simulink model "main"  (R2016b)
settings: Solver=FixedStepAuto  StartTime=0.0  StopTime=inf  FixedStep=Ts  MaxStep=0.2  RelTol=1e-2
undefined symbols (not defined in the file): checks, datetime, decyear, delta_e, deltae_degrees, deltafl_degrees, deltafr_degrees, deltar_degrees, deltat_1, deltat_2, deltat_3, deltat_4, deltat_5, Earth, F, ft, groundReaction, initialValues, juliandate, LD, leapyear, Light, m, MIL, Newton, Raphson, s, sigbuilder_block, Ts, WGS84
libraries: simulink x68, aerolibutil x17, aerolibtransform2 x15, simulink_extras x13, aerolibasang x5, aerolib6dofsys x5, aerolib6dof2 x4, aerolibwind2 x3, aerolibbdyn x3, vrlib x3, aerolibconvert2 x3, aerolibactuator x2
(part 1 of 10)
settings Model: Creator=Uxío  LastModifiedBy=sork9
settings DataIOCC: ReturnWorkspaceOutputs=on  ReturnWorkspaceOutputsName=spidata
settings OptimizationCC: EfficientMapNaN2IntZero=off  SimCompilerOptimization=on
settings DebuggingCC: ReadBeforeWriteMsg=DisableAll  WriteAfterWriteMsg=DisableAll  WriteAfterReadMsg=DisableAll  MultiTaskDSMMsg=none
settings HardwareCC: TargetBitPerPointer=64  TargetBitPerSizeT=64  TargetBitPerPtrDiffT=64  TargetLongLongMode=on  TargetIntDivRoundTo=Zero  TargetEndianess=LittleEndian  TargetWordSize=64  TargetHWDeviceType=MATLAB Host  ProdEqTarget=off
settings ModelReferenceCC: UpdateModelReferenceTargets=IfOutOfDate
settings SFSimCC: SFSimEcho=off
settings CodeAppCC: MaxIdLength=128
settings GRTTargetCC: TargetLangStandard=C89/C90 (ANSI)  CombineOutputUpdateFcns=off  GRTInterface=on
settings ConfigComp: PSAutoStubLUT=on

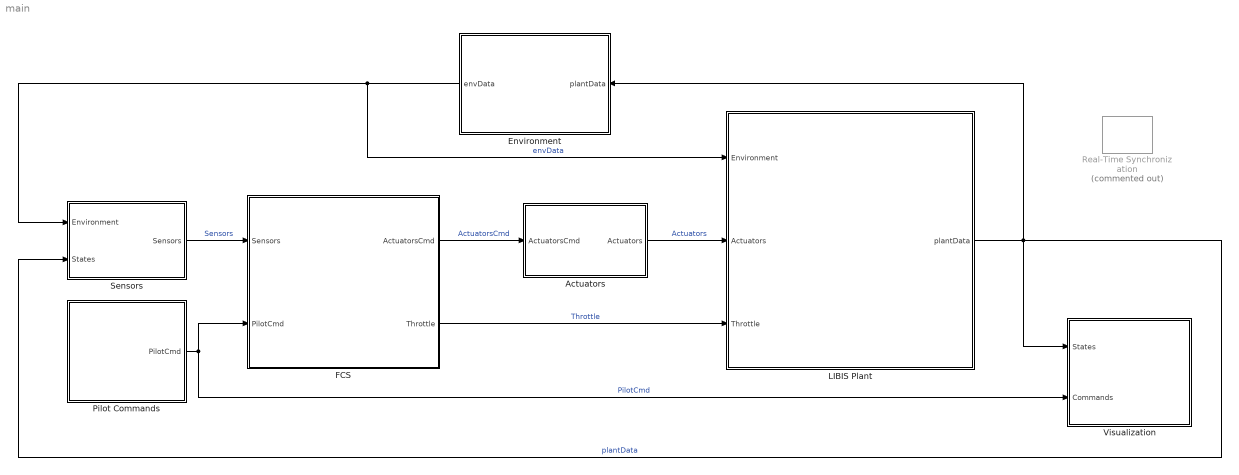
== system main ==
  Actuators : Subsystem  Variant=on
  Environment : Subsystem
      mask Display:
      | imageName='Wind.png';
      | currentPath=get_param(bdroot, 'FileName');
      | positions=strfind(currentPath,'\');
      | imagePath=strcat(currentPath(1:positions(end-1)),'graphics\',imageName);
      | image(imagePath);
  FCS : Subsystem
      mask Display:
      | imageName='FCS.png';
      | currentPath=get_param(bdroot, 'FileName');
      | positions=strfind(currentPath,'\');
      | imagePath=strcat(currentPath(1:positions(end-1)),'graphics\',imageName);
      | image(imagePath);
  LIBIS Plant : Subsystem
      mask Display:
      | imageName='LIBIS_Plant.jpg';
      | currentPath=get_param(bdroot, 'FileName');
      | positions=strfind(currentPath,'\');
      | imagePath=strcat(currentPath(1:positions(end-1)),'graphics\',imageName);
      | image(imagePath);
  Pilot Commands : Subsystem  VariantControl=Variants.Command==0
      mask Display:
      | imageName='Pilot.png';
      | currentPath=get_param(bdroot, 'FileName');
      | positions=strfind(currentPath,'\');
      | imagePath=strcat(currentPath(1:positions(end-1)),'graphics\',imageName);
      | image(imagePath);
  Real-Time Synchronization : sldrtlib/Real-Time Synchronization  Commented=on  SampleTime=Ts  MaxMissedTicks=25  ShowMissedTicks=off  YieldWhenWaiting=on
  Sensors : Subsystem  Variant=on
  Visualization : Subsystem
  wires:
  FCS/2(Throttle) -> LIBIS Plant/3(Throttle)  "Throttle"
  LIBIS Plant/1(plantData) -> Visualization/1(States), Sensors/2(States), Environment/1(plantData)  "plantData"
  Pilot Commands/1(PilotCmd) -> Visualization/2(Commands), FCS/2(PilotCmd)  "PilotCmd"
  Sensors/1(Sensors) -> FCS/1(Sensors)  "Sensors"
  Environment/1(envData) -> Sensors/1(Environment), LIBIS Plant/1(Environment)  "envData"
  FCS/1(ActuatorsCmd) -> Actuators/1(ActuatorsCmd)  "ActuatorsCmd"
  Actuators/1(Actuators) -> LIBIS Plant/2(Actuators)  "Actuators"

== system main/Actuators ==
  note: 1) Add Subsystem or Model blocks as valid variant choices.
      | 2) You cannot connect blocks at this level. At simulation, connectivity is automatically
      | determined, based on the active variant and port name matching.
  ActuatorsCmd : Inport  OutDataTypeStr=Bus: ActuatorsBus
  Feedthrough : Subsystem  VariantControl=actuatorsDynamics==0
  Linear 1st Order : Subsystem  VariantControl=actuatorsDynamics==1  mask{a=LD.Actuators.LFO.timeLag}
      mask prompts: a "Actuator Time Constant Inverse:"
  Linear 2nd Order : Subsystem  VariantControl=actuatorsDynamics==2
  Nonlinear 2nd Order : Subsystem  VariantControl=actuatorsDynamics==3
  Actuators : Outport  OutDataTypeStr=Bus: ActuatorsBus

== system main/Environment ==
  plantData : Inport  OutDataTypeStr=Bus: plantDataBus
  Bus Selector : BusSelector  OutputSignals=LLA.Altitude_m,X_ned,V_ned,Omega_body,CG,DCM_body_earth,LLA.Latitude_deg,LLA.Longitude_deg
  COESA Atmosphere Model : aerolibatmos2/COESA Atmosphere Model  units=Metric (MKS)  spec=1976 COESA-extended U.S. Standard Atmosphere  model=Profile  profile_var=High temperature  profile_percent=1%  profile_alt=5 km (16404 ft)  envelope_var=High temperature  envelope_percent=1%  action=Warning
  Clock : Clock
  Gravity in Earth Axes : Gain  Gain=[0 0 LD.Inertia.mass]  SaturateOnIntegerOverflow=on  OutDataTypeStr=Inherit: Same as input  ParamDataTypeStr=Inherit: Same as input
  Initial Decimal date : Constant  Value=decyear(datetime(initialValues.Date,'InputFormat','dd-MMM-yyyy hh:mm:ss'))
  Initial Julian  date : Constant  Value=juliandate(datetime(initialValues.Date,'InputFormat','dd-MMM-yyyy hh:mm:ss'))
  Math Function : Math  Operator=transpose  SaturateOnIntegerOverflow=on
  Mux : Mux  Inputs=3
  Reshape : Reshape
  Reshape1 : Reshape
  Reshape2 : Reshape
  Sum : Sum  Inputs=++|
  Sum1 : Sum  Inputs=|++
  Terrain : Subsystem
  To Body Axes : Product  Multiplication=Matrix(*)  SaturateOnIntegerOverflow=on  InputSameDT=on  OutDataTypeStr=Inherit: Same as first input
  "WGS84 Gravity Model " : aerolibgravity2/WGS84 Gravity Model   model=WGS84 Exact  units=Metric (MKS)  no_atmos=on  precessing=on  jd_loc=on  month=October  day=10  year=2004  no_centrifugal=on  action=Warning
  Wind Models : Subsystem
  World Magnetic Model 2015 : aerolibgravity2/World Magnetic Model 2015  units=Metric (MKS)  time_in=on  month=January  day=1  year=2015  action=Warning  h_out=off  dec_out=off  inc_out=off  ti_out=off
  envDataBus : BusCreator  Inputs='h_ground','Fground','Mground','windVelocity','windOmega','T','a','P','AirDensity','Fgravity','Gravity_ned','MagneticField_ned'  OutDataTypeStr=Bus: envDataBus  NonVirtualBus=on
  kclock : Gain  Gain=1/(60*60*24*(365 + leapyear(floor(decyear(initialValues.Date,'dd-mmm-yyyy')))))
  envData : Outport  OutDataTypeStr=Bus: envDataBus  InitialOutput=0
  wires:
  [Altitude] -> COESA Atmosphere Model/1
  Bus Selector/6 -> To Body Axes/1, Wind Models/3(DCM_be), Terrain/5(DCM_body_earth)  "<DCM_body_earth>"
  Bus Selector/7 -> World Magnetic Model 2015/2, Mux/1  "<Latitude_deg>"
  Bus Selector/3 -> Wind Models/1(Ve), Terrain/2(Ve)  "<V_ned>"
  [Altitude] -> Mux/3
  envDataBus/1 -> envData/1  "envData"
  To Body Axes/1 -> Reshape/1  "Fg"
  Wind Models/2(windOmega) -> envDataBus/5  "windOmega"
  Bus Selector/2 -> Terrain/1(Xe)  "<X_ned>"
  COESA Atmosphere Model/3 -> envDataBus/8  "P"
  COESA Atmosphere Model/2 -> envDataBus/7  "a"
  Wind Models/1(windVelocity) -> envDataBus/4  "windVelocity"
  [Altitude] -> Wind Models/2(Altitude)
  COESA Atmosphere Model/1 -> envDataBus/6  "T"
  COESA Atmosphere Model/4 -> envDataBus/9  "AirDensity"
  Terrain/1(hground) -> envDataBus/1  "h_ground"
  Bus Selector/1 -> [Altitude]  "<Altitude_m>"
  Gravity in Earth Axes/1 -> Math Function/1
  Math Function/1 -> To Body Axes/2
  Reshape/1 -> envDataBus/10  "Fgravity"
  Reshape1/1 -> envDataBus/2  "Fground"
  plantData/1 -> Bus Selector/1
  Bus Selector/5 -> Terrain/4("CG ")  "<CG>"
  Reshape2/1 -> envDataBus/3  "Mground"
  Bus Selector/4 -> Terrain/3("Omega_body ")  "<Omega_body>"
  Terrain/3(Mground) -> Reshape2/1
  Terrain/2(Fground) -> Reshape1/1
  World Magnetic Model 2015/1 -> envDataBus/12  "MagneticField_ned"
  Clock/1 -> kclock/1
  Initial Decimal date/1 -> Sum/2
  Sum/1 -> World Magnetic Model 2015/4
  [Altitude] -> World Magnetic Model 2015/1
  Bus Selector/8 -> World Magnetic Model 2015/3, Mux/2  "<Longitude_deg>"
  "WGS84 Gravity Model "/1 -> Gravity in Earth Axes/1, envDataBus/11  "Gravity_ned"
  Mux/1 -> "WGS84 Gravity Model "/1
  Initial Julian  date/1 -> Sum1/1
  Sum1/1 -> "WGS84 Gravity Model "/2
  kclock/1 -> Sum/1, Sum1/2

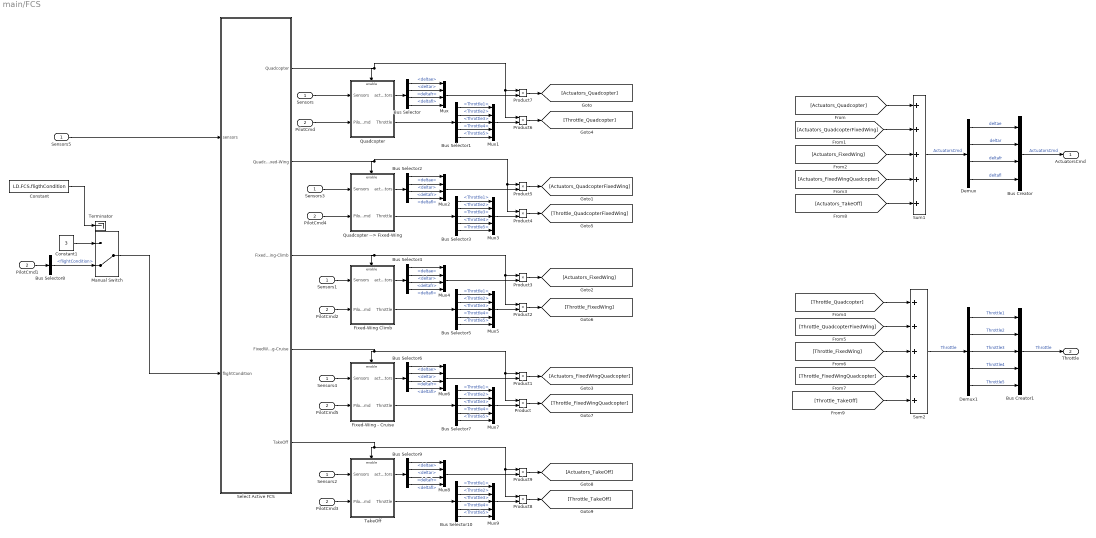
== system main/FCS ==
  Sensors : Inport  OutDataTypeStr=Bus: SensorsBus
  PilotCmd : Inport  Port=2  OutDataTypeStr=Bus: CommandBus
  Bus Creator : BusCreator  Inputs='deltae','deltar','deltafr','deltafl'  OutDataTypeStr=Bus: ActuatorsBus  NonVirtualBus=on
  Bus Creator1 : BusCreator  Inputs='Throttle1','Throttle2','Throttle3','Throttle4','Throttle5'  OutDataTypeStr=Bus: ThrottleBus  NonVirtualBus=on
  Bus Selector{,2,4,6,9} (5 alike) : BusSelector  OutputSignals=deltae,deltar,deltafr,deltafl
  Bus Selector{1,3,5,7,10} (5 alike) : BusSelector  OutputSignals=Throttle1,Throttle2,Throttle3,Throttle4,Throttle5
  Bus Selector8 : BusSelector  OutputSignals=flightCondition
  Constant : Constant  Value=LD.FCS.fligthCondition
  Constant1 : Constant  Value=3
  Demux : Demux
  Demux1 : Demux  Outputs=5
  Fixed-Wing - Cruise : Subsystem  TreatAsAtomicUnit=on
  Fixed-Wing Climb : Subsystem  TreatAsAtomicUnit=on
  Manual Switch : ManualSwitch  CurrentSetting=0
  Mux{,2,4,6,8} (5 alike) : Mux
  Mux{1,3,5,7,9} (5 alike) : Mux  Inputs=5
  PilotCmd{1..5} (5 alike) : InportShadow  Port=2  OutDataTypeStr=Bus: CommandBus
  Product{,1..9} (10 alike) : Product
  Quadcopter : Subsystem  TreatAsAtomicUnit=on
  Quadcopter --> Fixed-Wing : Subsystem  TreatAsAtomicUnit=on
  Select Active FCS : Subsystem
  Sensors{1..5} (5 alike) : InportShadow  OutDataTypeStr=Bus: SensorsBus
  Sum1 : Sum  Inputs=+++++
  Sum2 : Sum  Inputs=+++++
  TakeOff : Subsystem  TreatAsAtomicUnit=on
  Terminator : Terminator
  ActuatorsCmd : Outport  OutDataTypeStr=Bus: ActuatorsBus
  Throttle : Outport  Port=2  OutDataTypeStr=Bus: ThrottleBus
  wires:
  Quadcopter/1(actuators) -> Bus Selector/1
  Quadcopter --> Fixed-Wing/1(actuators) -> Bus Selector2/1
  Fixed-Wing - Cruise/1(actuators) -> Bus Selector6/1
  [Actuators_Quadcopter] -> Sum1/1
  [Actuators_QuadcopterFixedWing] -> Sum1/2
  [Actuators_FixedWingQuadcopter] -> Sum1/4
  [Actuators_FixedWing] -> Sum1/3
  [Throttle_Quadcopter] -> Sum2/1
  [Throttle_QuadcopterFixedWing] -> Sum2/2
  [Throttle_FixedWing] -> Sum2/3
  [Throttle_FixedWingQuadcopter] -> Sum2/4
  PilotCmd/1 -> Quadcopter/2(PilotCmd)
  Bus Creator/1 -> ActuatorsCmd/1  "ActuatorsCmd"
  Sum1/1 -> Demux/1  "ActuatorsCmd"
  Demux/1 -> Bus Creator/1  "deltae"
  Demux/4 -> Bus Creator/4  "deltafl"
  Demux/3 -> Bus Creator/3  "deltafr"
  Demux/2 -> Bus Creator/2  "deltar"
  Bus Creator1/1 -> Throttle/1  "Throttle"
  Sum2/1 -> Demux1/1  "Throttle"
  Demux1/1 -> Bus Creator1/1  "Throttle1"
  Demux1/4 -> Bus Creator1/4  "Throttle4"
  Demux1/3 -> Bus Creator1/3  "Throttle3"
  Demux1/2 -> Bus Creator1/2  "Throttle2"
  Demux1/5 -> Bus Creator1/5  "Throttle5"
  Bus Selector/1 -> Mux/1  "<deltae>"
  Bus Selector/2 -> Mux/2  "<deltar>"
  Bus Selector/3 -> Mux/3  "<deltafr>"
  Bus Selector/4 -> Mux/4  "<deltafl>"
  Quadcopter/2(Throttle) -> Bus Selector1/1
  Bus Selector1/1 -> Mux1/1  "<Throttle1>"
  Bus Selector1/2 -> Mux1/2  "<Throttle2>"
  Bus Selector1/3 -> Mux1/3  "<Throttle3>"
  Bus Selector1/4 -> Mux1/4  "<Throttle4>"
  Bus Selector1/5 -> Mux1/5  "<Throttle5>"
  Bus Selector2/1 -> Mux2/1  "<deltae>"
  Bus Selector2/2 -> Mux2/2  "<deltar>"
  Bus Selector2/3 -> Mux2/3  "<deltafr>"
  Bus Selector2/4 -> Mux2/4  "<deltafl>"
  Quadcopter --> Fixed-Wing/2(Throttle) -> Bus Selector3/1
  Bus Selector3/1 -> Mux3/1  "<Throttle1>"
  Bus Selector3/2 -> Mux3/2  "<Throttle2>"
  Bus Selector3/3 -> Mux3/3  "<Throttle3>"
  Bus Selector3/4 -> Mux3/4  "<Throttle4>"
  Bus Selector3/5 -> Mux3/5  "<Throttle5>"
  Bus Selector4/1 -> Mux4/1  "<deltae>"
  Bus Selector4/2 -> Mux4/2  "<deltar>"
  Bus Selector4/3 -> Mux4/3  "<deltafr>"
  Bus Selector4/4 -> Mux4/4  "<deltafl>"
  Fixed-Wing Climb/2(Throttle) -> Bus Selector5/1
  Bus Selector5/1 -> Mux5/1  "<Throttle1>"
  Bus Selector5/2 -> Mux5/2  "<Throttle2>"
  Bus Selector5/3 -> Mux5/3  "<Throttle3>"
  Bus Selector5/4 -> Mux5/4  "<Throttle4>"
  Bus Selector5/5 -> Mux5/5  "<Throttle5>"
  Bus Selector6/1 -> Mux6/1  "<deltae>"
  Bus Selector6/2 -> Mux6/2  "<deltar>"
  Bus Selector6/3 -> Mux6/3  "<deltafr>"
  Bus Selector6/4 -> Mux6/4  "<deltafl>"
  Fixed-Wing - Cruise/2(Throttle) -> Bus Selector7/1
  Bus Selector7/1 -> Mux7/1  "<Throttle1>"
  Bus Selector7/2 -> Mux7/2  "<Throttle2>"
  Bus Selector7/3 -> Mux7/3  "<Throttle3>"
  Bus Selector7/4 -> Mux7/4  "<Throttle4>"
  Bus Selector7/5 -> Mux7/5  "<Throttle5>"
  Constant/1 -> Terminator/1
  PilotCmd1/1 -> Bus Selector8/1
  Bus Selector8/1 -> Manual Switch/2  "<flightCondition>"
  Manual Switch/1 -> Select Active FCS/2(flightCondition)
  Mux7/1 -> Product/2
  Mux6/1 -> Product1/2
  Select Active FCS/4(FixedWing-Cruise) -> Fixed-Wing - Cruise/Enable, Product1/1, Product/1
  Product/1 -> [Throttle_FixedWingQuadcopter]
  Product1/1 -> [Actuators_FixedWingQuadcopter]
  Mux5/1 -> Product2/2
  Mux4/1 -> Product3/2
  Select Active FCS/3(FixedWing-Climb) -> Fixed-Wing Climb/Enable, Product2/1, Product3/1
  Mux3/1 -> Product4/2
  Mux2/1 -> Product5/2
  Select Active FCS/2(Quadcopter-->Fixed-Wing) -> Product5/1, Product4/1, Quadcopter --> Fixed-Wing/Enable
  Mux1/1 -> Product6/2
  Mux/1 -> Product7/2
  Select Active FCS/1(Quadcopter) -> Product6/1, Product7/1, Quadcopter/Enable
  Product7/1 -> [Actuators_Quadcopter]
  Product6/1 -> [Throttle_Quadcopter]
  Product5/1 -> [Actuators_QuadcopterFixedWing]
  Product4/1 -> [Throttle_QuadcopterFixedWing]
  Product3/1 -> [Actuators_FixedWing]
  Product2/1 -> [Throttle_FixedWing]
  Fixed-Wing Climb/1(actuators) -> Bus Selector4/1
  Sensors1/1 -> Fixed-Wing Climb/1(Sensors)
  PilotCmd2/1 -> Fixed-Wing Climb/2(PilotCmd)
  Bus Selector9/1 -> Mux8/1  "<deltae>"
  Bus Selector9/2 -> Mux8/2  "<deltar>"
  Bus Selector9/3 -> Mux8/3  "<deltafr>"
  Bus Selector9/4 -> Mux8/4  "<deltafl>"
  TakeOff/2(Throttle) -> Bus Selector10/1
  Bus Selector10/1 -> Mux9/1  "<Throttle1>"
  Bus Selector10/2 -> Mux9/2  "<Throttle2>"
  Bus Selector10/3 -> Mux9/3  "<Throttle3>"
  Bus Selector10/4 -> Mux9/4  "<Throttle4>"
  Bus Selector10/5 -> Mux9/5  "<Throttle5>"
  Mux9/1 -> Product8/2
  Mux8/1 -> Product9/2
  Select Active FCS/5(TakeOff) -> TakeOff/Enable, Product8/1, Product9/1
  Product9/1 -> [Actuators_TakeOff]
  Product8/1 -> [Throttle_TakeOff]
  TakeOff/1(actuators) -> Bus Selector9/1
  Sensors2/1 -> TakeOff/1(Sensors)
  PilotCmd3/1 -> TakeOff/2(PilotCmd)
  [Actuators_TakeOff] -> Sum1/5
  [Throttle_TakeOff] -> Sum2/5
  Constant1/1 -> Manual Switch/1
  Sensors/1 -> Quadcopter/1(Sensors)
  PilotCmd4/1 -> Quadcopter --> Fixed-Wing/2(PilotCmd)
  Sensors3/1 -> Quadcopter --> Fixed-Wing/1(Sensors)
  PilotCmd5/1 -> Fixed-Wing - Cruise/2(PilotCmd)
  Sensors4/1 -> Fixed-Wing - Cruise/1(Sensors)
  Sensors5/1 -> Select Active FCS/1(sensors)

== system main/LIBIS Plant ==
  Environment : Inport  OutDataTypeStr=Bus: envDataBus
  Actuators : Inport  Port=2  OutDataTypeStr=Bus: ActuatorsBus
  Throttle : Inport  Port=3  OutDataTypeStr=Bus: ThrottleBus
  Aerodynamics : Subsystem
  Bus Selector : BusSelector  OutputSignals=Fgravity,Fground,Mground
  Bus Selector1 : BusSelector  OutputSignals=windVelocity
  Constant : Constant  Value=initialValues.href
  "Custom Variable Mass 6DOF (Euler Angles) " : Subsystem  mask(6DOF EoM (Body Axis)){units=Metric (MKS), mtype=Custom Variable, rep=Euler Angles, xme_0=[initialValues.Xe0 initialValues.Ye0 initialValues.Ze0], Vm_0=[initialValues.u0 initialValues.v0 initialValues.w0], eul_0=[initialValues.roll0 initialValues.pitch0 initialValues.yaw0], pm_0=[initialValues.p0 initialValues.q0 initialValues.r0], mass_0=1.0, mass_e=0.5, mass_f=2.0, inertia=eye(3), inertia_e=eye(3), inertia_f=2*eye(3), k_quat=1.0, vre_flag=on}
      mask prompts: units "aeroblks:aeroblk6dofbody:block6DOFEoMBodyAxisParamUnits"; mtype "aeroblks:aeroblk6dofbody:block6DOFEoMBodyAxisParamMasstype"; rep "aeroblks:aeroblk6dofbody:block6DOFEoMBodyAxisParamRepresentation"; xme_0 "aeroblks:aeroblk6dofbody:block6DOFEoMBodyAxisParamInitialpositionininertialaxesXeYeZe"; Vm_0 "aeroblks:aeroblk6dofbody:block6DOFEoMBodyAxisParamInitialvelocityinbodyaxesUvw"; eul_0 "aeroblks:aeroblk6dofbody:block6DOFEoMBodyAxisParamInitialEulerorientationrollpitchyaw"; pm_0 "aeroblks:aeroblk6dofbody:block6DOFEoMBodyAxisParamInitialbodyrotationratespqr"; mass_0 "aeroblks:aeroblk6dofbody:block6DOFEoMBodyAxisParamInitialmass"; mass_e "aeroblks:aeroblk6dofbody:block6DOFEoMBodyAxisParamEmptymass"; mass_f "aeroblks:aeroblk6dofbody:block6DOFEoMBodyAxisParamFullmass"; inertia "aeroblks:aeroblk6dofbody:block6DOFEoMBodyAxisParamInertia"; inertia_e "aeroblks:aeroblk6dofbody:block6DOFEoMBodyAxisParamEmptyinertiamatrix"; inertia_f "aeroblks:aeroblk6dofbody:block6DOFEoMBodyAxisParamFullinertiamatrix"; k_quat "aeroblks:aeroblk6dofbody:block6DOFEoMBodyAxisParamGainforquaternionnormalization"; vre_flag "aeroblks:aeroblk6dofbody:block6DOFEoMBodyAxisParamIncludemassflowrelativevelocity"
      mask help: aeroblks:aeroblk6dofbody:block6DOFEoMBodyAxisDesc
      mask init:
      | ports=aeroicon('aeroblk6dofbody','icon');
      mask Help: eval('asbhelp(''custom_variable_mass_sixdof_euler_angles'')');
      mask TypeOptions units: aeroblks:aeroblk6dofbody:block6DOFEoMBodyAxisParamComboMetricMKS | aeroblks:aeroblk6dofbody:block6DOFEoMBodyAxisParamComboEnglishVelocityinfts | aeroblks:aeroblk6dofbody:block6DOFEoMBodyAxisParamComboEnglishVelocityinkts
      mask TypeOptions mtype: aeroblks:aeroblk6dofbody:block6DOFEoMBodyAxisParamComboFixed | aeroblks:aeroblk6dofbody:block6DOFEoMBodyAxisParamComboSimpleVariable | aeroblks:aeroblk6dofbody:block6DOFEoMBodyAxisParamComboCustomVariable
      mask Callback mtype: aeroicon('aeroblk6dofbody');
      mask TypeOptions rep: aeroblks:aeroblk6dofbody:block6DOFEoMBodyAxisParamComboEulerAngles | aeroblks:aeroblk6dofbody:block6DOFEoMBodyAxisParamComboQuaternion
      mask Callback rep: aeroicon('aeroblk6dofbody');
      mask Display:
      | port_label(ports(1).type,ports(1).port,ports(1).txt,'texmode','on');
      | port_label(ports(2).type,ports(2).port,ports(2).txt,'texmode','on');
      | port_label(ports(3).type,ports(3).port,ports(3).txt,'texmode','on');
      | port_label(ports(4).type,ports(4).port,ports(4).txt,'texmode','on');
      | port_label(ports(5).type,ports(5).port,ports(5).txt,'texmode','on');
      | port_label(ports(6).type,ports(6).port,ports(6).txt,'texmode','on');
      | port_label(ports(7).type,ports(7).port,ports(7).txt,'texmode','on');
      | port_label(ports(8).type,ports(8).port,ports(8).txt,'texmode','on');
      | port_label(ports(9).type,ports(9).port,ports(9).txt,'texmode','on');
      | port_label(ports(10).type,ports(10).port,ports(10).txt,'texmode','on');
      | port_label(ports(11).type,ports(11).port,ports(11).txt,'texmode','on');
      | port_label(ports(12).type,ports(12).port,ports(12).txt,'texmode','on');
      | port_label(ports(13).type,ports(13).port,ports(13).txt,'texmode','on');
      | port_label(ports(14).type,ports(14).port,ports(14).txt,'texmode','on');
      | port_label(ports(15).type,ports(15).port,ports(15).txt,'texmode','on');
      | port_label(ports(16).type,ports(16).port,ports(16).txt,'texmode','on');
      | [x y xp yp highstr lowstr maxy miny]=aeroimage('sixdofbody',gcbh);
      | text(0.5,maxy+0.065,highstr{:},'horizontalAlignment','center')
      | text(0.5,miny-0.06,lowstr{:},'horizontalAlignment','center')
      | plot(x,y);
      | patch(xp, yp);
  Demux1 : Demux  Outputs=3
  Demux2 : Demux  Outputs=2
  Demux3 : Demux  Outputs=3
  Derivative : Derivative
  Derivative1 : Derivative
  EulerBus : BusCreator  Inputs='phi','theta','psi'  OutDataTypeStr=Bus: EulerBus  NonVirtualBus=on
  Flat Earth to LLA : aerolibtransform2/Flat Earth to LLA  units=Metric (MKS)  ptype=Earth (WGS84)  F=1/298.257223563  R=6378137  LL0=initialValues.LatLong0  psi=initialValues.heading0
  IC : InitialCondition  Value=[0 0 0]
  IC1 : InitialCondition  Value=[0 0 0]
  IC10 : InitialCondition  Value=[initialValues.D,0,0]
  IC11 : InitialCondition  Value=[initialValues.uned0 initialValues.vned0 initialValues.wned0]
  IC12 : InitialCondition  Value=[0 0 -initialValues.href]
  IC13 : InitialCondition  Value=[-initialValues.D,0,-initialValues.L]
  IC2 : InitialCondition  Value=[initialValues.roll0, initialValues.pitch0, initialValues.yaw0]
  IC3 : InitialCondition  Value=[initialValues.p0 initialValues.q0 initialValues.r0]
  IC4 : InitialCondition  Value=[initialValues.Xe0 initialValues.Ye0 initialValues.Ze0]
  IC5 : InitialCondition  Value=[initialValues.u0 initialValues.v0 initialValues.w0]
  IC6 : InitialCondition  Value=[initialValues.Fx0 initialValues.Fy0 initialValues.Fz0]
  IC7 : InitialCondition  Value=initialValues.alpha_wb
  IC8 : InitialCondition  Value=0
  IC9 : InitialCondition  Value=[initialValues.Mx0 initialValues.My0 initialValues.Mz0]
  "Incidence, Sideslip" : Subsystem
  Inertia Block : Subsystem
      mask Display:
      | imageName='Moment_of_inertia.png';
      | currentPath=get_param(bdroot, 'FileName');
      | positions=strfind(currentPath,'\');
      | imagePath=strcat(currentPath(1:positions(end-1)),'graphics\',imageName);
      | image(imagePath);
  LLABus : BusCreator  Inputs='Latitude_deg','Longitude_deg','Altitude_m'  OutDataTypeStr=Bus: LLABus  NonVirtualBus=on
  OmegaBus : BusCreator  Inputs='p','q','r'  OutDataTypeStr=Bus: OmegaBus  NonVirtualBus=on
  Propulsion : Subsystem
  Rate Limiter : RateLimiter  RisingSlewLimit=100  FallingSlewLimit=-100  SampleTimeMode=inherited
  Rate Limiter1 : RateLimiter  RisingSlewLimit=100  FallingSlewLimit=-100  SampleTimeMode=inherited
  Subsystem : Subsystem  Commented=on
  Sum : Sum  Inputs=++++
  Sum1 : Sum  Inputs=||+++
  Sum2 : Sum  Inputs=+-|
  Terminator1 : Terminator
  TransferFunction : Subsystem
  TransferFunctions : Subsystem
  "alpha_dot, beta_dot" : Subsystem  Commented=on
  envData1 : InportShadow  OutDataTypeStr=Bus: envDataBus
  plantDataBus : BusCreator  Inputs='LLA','V_ned','X_ned','Euler','DCM_body_earth','V_body','Omega_body','dOmega_body','Accel_body','alpha','beta','alpha_dot','beta_dot','CG','remainingCapacity'  OutDataTypeStr=Bus: plantDataBus  NonVirtualBus=on
  plantData : Outport  OutDataTypeStr=Bus: plantDataBus
  wires:
  Inertia Block/4(I (kg-m^2)) -> "Custom Variable Mass 6DOF (Euler Angles) "/6(I)
  plantDataBus/1 -> Propulsion/3(plantData), Aerodynamics/1(plantData), plantData/1  "plantData"
  Flat Earth to LLA/2 -> LLABus/3  "Altitude_m"
  "Custom Variable Mass 6DOF (Euler Angles) "/2(Xe) -> IC12/1, IC4/1  "X_ned"
  "Custom Variable Mass 6DOF (Euler Angles) "/3(Euler) -> IC2/1  "Euler"
  EulerBus/1 -> plantDataBus/4  "Euler"
  Flat Earth to LLA/1 -> Demux2/1
  Demux2/1 -> LLABus/1  "Latitude_deg"
  Inertia Block/2(m (kg)) -> "Custom Variable Mass 6DOF (Euler Angles) "/4(mass)
  Inertia Block/5(Vre (m/s)) -> "Custom Variable Mass 6DOF (Euler Angles) "/7(Vre)
  "Custom Variable Mass 6DOF (Euler Angles) "/5(Vb) -> IC5/1  "V_body"
  Inertia Block/7(dCG/dt) -> Terminator1/1
  [CG] -> plantDataBus/14  "CG"
  "Custom Variable Mass 6DOF (Euler Angles) "/4(DCM) -> plantDataBus/5  "DCM_body_earth"
  Inertia Block/3(dI/dt (kg-m^2/s)) -> "Custom Variable Mass 6DOF (Euler Angles) "/5(I_dot)
  LLABus/1 -> plantDataBus/1  "LLA"
  "Incidence, Sideslip"/1(Alpha) -> IC7/1  "alpha"
  Demux3/1 -> EulerBus/1  "phi"
  Demux3/3 -> EulerBus/3  "psi"
  Inertia Block/6(CG) -> [CG]
  Inertia Block/1(dm/dt (kg/s)) -> "Custom Variable Mass 6DOF (Euler Angles) "/3(m_dot)
  Constant/1 -> Flat Earth to LLA/2
  Demux2/2 -> LLABus/2  "Longitude_deg"
  "Incidence, Sideslip"/2(Beta) -> IC8/1  "beta"
  Demux3/2 -> EulerBus/2  "theta"
  "Custom Variable Mass 6DOF (Euler Angles) "/1(Ve) -> IC11/1  "V_ned"
  OmegaBus/1 -> plantDataBus/7  "Omega_body"
  "Custom Variable Mass 6DOF (Euler Angles) "/6(p,q,r) -> IC3/1  "Omega_body"
  Demux1/2 -> OmegaBus/2  "q"
  Demux1/1 -> OmegaBus/1  "p"
  Demux1/3 -> OmegaBus/3  "r"
  Actuators/1 -> Aerodynamics/2(Actuators)  "Actuators"
  Throttle/1 -> Propulsion/2(Throttle)  "Throttle"
  Propulsion/3(remainingCapacity) -> [remainingCapacity]
  [remainingCapacity] -> plantDataBus/15  "remainingCapacity"
  Propulsion/1(Total_Thrust) -> IC10/1  "Fthrust_body"
  Environment/1 -> Propulsion/1(envData), Bus Selector/1, Aerodynamics/3(envData)
  IC4/1 -> Flat Earth to LLA/1
  IC5/1 -> plantDataBus/6, Sum2/1  "V_body"
  IC3/1 -> Demux1/1  "Omega_body"
  IC2/1 -> Demux3/1
  Bus Selector/1 -> Sum/2  "<Fgravity>"
  IC7/1 -> plantDataBus/10, Derivative/1  "alpha"
  envData1/1 -> Bus Selector1/1
  Bus Selector/2 -> Sum/3  "<Fground>"
  Bus Selector1/1 -> TransferFunction/1(In1)  "<windVelocity>"
  Sum2/1 -> "Incidence, Sideslip"/1("u, v, w")  "Vaero"
  "Custom Variable Mass 6DOF (Euler Angles) "/7(pdot,qdot,rdot) -> IC/1  "dOmega_body"
  "Custom Variable Mass 6DOF (Euler Angles) "/8(Ab) -> IC1/1  "Accel_body"
  IC8/1 -> Derivative1/1, plantDataBus/11  "beta"
  Sum1/1 -> IC9/1
  Sum/1 -> IC6/1
  IC6/1 -> "Custom Variable Mass 6DOF (Euler Angles) "/1(Forces)  "Fxyz"
  IC9/1 -> "Custom Variable Mass 6DOF (Euler Angles) "/2(Moments)  "Mxyz"
  IC/1 -> TransferFunctions/1(In1)  "dOmega_body"
  IC1/1 -> TransferFunctions/2(In2)  "Accel_body"
  TransferFunctions/1(Out1) -> plantDataBus/8  "dOmega_body"
  TransferFunctions/2(Out2) -> plantDataBus/9  "Accel_body"
  IC11/1 -> plantDataBus/2  "V_ned"
  IC12/1 -> plantDataBus/3  "X_ned"
  Rate Limiter1/1 -> plantDataBus/13  "beta_dot"
  TransferFunction/1(Out1) -> Sum2/2  "windVelocity"
  Rate Limiter/1 -> plantDataBus/12  "alpha_dot"
  Aerodynamics/2(Mbody) -> Sum1/1  "Maero"
  Aerodynamics/1(Fbody) -> IC13/1  "Faero_body"
  Bus Selector/3 -> Sum1/2  "<Mground>"
  Propulsion/2(Total_Thrust_Moment) -> Sum1/3  "Mthrust"
  Derivative/1 -> Rate Limiter/1
  Derivative1/1 -> Rate Limiter1/1
  IC13/1 -> Sum/1
  IC10/1 -> Sum/4

== system main/Pilot Commands ==
  note: Ejemplos de maniobras:
      |
      | 1.Despegue quadrotor - transición - crucero:
      | Para realizar esta maniobra debe iniciarse la simulación desde el modo de control
      | ’Quadrotor’ y con el control por joystick desactivado. La aeronave volará hasta el
      | punto especificado por defecto en ’Comanded position in Earth axis’ [10,2, 10]. Una
      | vez estabilizada en este punto, debe seleccionarse el modo ’Transition’. Al alcanzar
      | la velocidad de seguridad para el ascenso, la aeronave entrará automáticamente en
      | modo ’Climb’.
      | Cuando la aeronave se encuentre a una altura superior a la del crucero elegido,
      | se activará el modo ’Cruise’ y se introducirá la altura de crucero en el campo
      | ’Comanded altitude’.
      | La maniobra puede realizarse de manera similar con el joystick activado, teniendo
      | un control más directo sobre el estado de la aeronave en todas las fases.
      |
      | 2. Despegue ala fija - ascenso - crucero:
      | Para realizar esta maniobra debe iniciarse la simulación desde el modo de control
      | ’Take-off’. Cuando la aeronave despegue del suelo y tome cierta altura de seguridad,
      | debe cambiarse al modo ’Climb, lo que permitirá ascender hasta régimen de crucero.
      | Una vez alcanzada la altura objetivo, se activará el modo ’Cruise’ y se considera
      | finalizada la maniobra
  note: Comands control panel
  note: Control mode selector
  note: Enable joystick:
  note: Comanded position in Earth axis (m)
  note: Comanded altitude (m)
  note: Signal builder
  " " : Subsystem  DialogController=hmiCreateDDGDialog  IsWebBlock=on  mask(MWDashboardBlock){webBlockId=8cf82eb4-b282-4f0c-ab68-3c14940a8c65, webBlockType=discreteknob, ShowInLibBrowser=on, ShowInitialText=on, HMISrcModelName=main}
      mask prompts: webBlockId "WebBlock Id"; webBlockType "WebBlock Type"; HMISrcModelName "Source Model"
      mask help: SimulinkHMI:dialogs:DiscreteKnobDialogDesc
      mask Help: helpview([docroot '/mapfiles/simulink.map'], 'hmi_rotary_switch')
      mask Display:
      | model = bdroot(gcb);
      | if strcmp(get_param(model,'BlockDiagramType'), 'library')
      |     image([(matlabroot) '/toolbox/simulink/hmi/icons/DiscreteKnob.png']);
      | end
  " " : Subsystem  DialogController=hmiCreateDDGDialog  IsWebBlock=on  mask(MWDashboardBlock){webBlockId=d8a0ce64-6f29-4953-bda1-52b346d7ee10, webBlockType=discreteknob, ShowInLibBrowser=on, ShowInitialText=on, HMISrcModelName=main}
      mask prompts: webBlockId "WebBlock Id"; webBlockType "WebBlock Type"; HMISrcModelName "Source Model"
      mask help: SimulinkHMI:dialogs:DiscreteKnobDialogDesc
      mask Help: helpview([docroot '/mapfiles/simulink.map'], 'hmi_rotary_switch')
      mask Display:
      | model = bdroot(gcb);
      | if strcmp(get_param(model,'BlockDiagramType'), 'library')
      |     image([(matlabroot) '/toolbox/simulink/hmi/icons/DiscreteKnob.png']);
      | end
  0 : Constant  Value=[10,2,10]
  Airspeed Indicator1 : Subsystem  DialogController=aeroblksHMICreateDDGDialog  IsWebBlock=on  mask(MWDashboardBlock){webBlockId=4a322002-ac4b-4e2d-b04c-dccf105437e0, webBlockType=airspeedindicator, ShowInLibBrowser=on, ShowInitialText=on, HMISrcModelName=main}
      mask prompts: webBlockId "WebBlock Id"; webBlockType "WebBlock Type"; HMISrcModelName "Source Model"
      mask help: aeroblksHMI:aeroblkhmi:AirspeedIndicatorDialogDesc
      mask Help: eval('asbhmihelp(''airspeedindicator'')');
      mask Display:
      | if strcmp(get_param(bdroot(gcb),'BlockDiagramType'), 'library')
      |  image([(matlabroot) '/toolbox/aeroblks/aeroblks/hmi/icons/AirspeedIndicatorIcon.svg'])
      | end
  Altimeter1 : Subsystem  DialogController=aeroblksHMICreateDDGDialog  IsWebBlock=on  mask(MWDashboardBlock){webBlockId=7e3cc476-3120-44dd-a294-1a07c20b6fda, webBlockType=altimeter, ShowInLibBrowser=on, ShowInitialText=on, HMISrcModelName=main}
      mask prompts: webBlockId "WebBlock Id"; webBlockType "WebBlock Type"; HMISrcModelName "Source Model"
      mask help: aeroblksHMI:aeroblkhmi:AltimeterDialogDesc
      mask Help: eval('asbhmihelp(''altimeter'')');
      mask Display:
      | if strcmp(get_param(bdroot(gcb),'BlockDiagramType'), 'library')
      |  image([(matlabroot) '/toolbox/aeroblks/aeroblks/hmi/icons/AltimeterIcon.svg'])
      | end
  Artificial Horizon1 : Subsystem  DialogController=aeroblksHMICreateDDGDialog  IsWebBlock=on  mask(MWDashboardBlock){webBlockId=74ab2c84-f67f-420d-bc53-b4d2b583d9bb, webBlockType=artificialhorizon, ShowInLibBrowser=on, ShowInitialText=on, HMISrcModelName=main}
      mask prompts: webBlockId "WebBlock Id"; webBlockType "WebBlock Type"; HMISrcModelName "Source Model"
      mask help: aeroblksHMI:aeroblkhmi:ArtificialHorizonDialogDesc
      mask Help: eval('asbhmihelp(''artificialhorizon'')');
      mask Display:
      | if strcmp(get_param(bdroot(gcb),'BlockDiagramType'), 'library')
      |  image([(matlabroot) '/toolbox/aeroblks/aeroblks/hmi/icons/ArtificialHorizonIcon.svg'])
      | end
  Bus Creator : BusCreator  Inputs='roll_cmd','pitch_cmd','yaw_cmd','altitude_cmd','Throttle1_cmd','flightCondition','Position_cmd','joystickEnabled'  OutDataTypeStr=Bus: CommandBus  NonVirtualBus=on
  Bus Creator1 : BusCreator  Inputs='roll_cmd','pitch_cmd','yaw_cmd','altitude_cmd','Throttle1_cmd','flightCondition','Position_cmd','joystickEnabled'  OutDataTypeStr=Bus: CommandBus  NonVirtualBus=on
  Buttons to Switches : Subsystem
  Climb Rate Indicator1 : Subsystem  DialogController=aeroblksHMICreateDDGDialog  IsWebBlock=on  mask(MWDashboardBlock){webBlockId=0e57c45c-8156-4b51-9f50-a7e28d9659ef, webBlockType=climbindicator, ShowInLibBrowser=on, ShowInitialText=on, HMISrcModelName=main}
      mask prompts: webBlockId "WebBlock Id"; webBlockType "WebBlock Type"; HMISrcModelName "Source Model"
      mask help: aeroblksHMI:aeroblkhmi:ClimbIndicatorDialogDesc
      mask Help: eval('asbhmihelp(''climbindicator'')');
      mask Display:
      | if strcmp(get_param(bdroot(gcb),'BlockDiagramType'), 'library')
      |  image([(matlabroot) '/toolbox/aeroblks/aeroblks/hmi/icons/ClimbIndicatorIcon.svg'])
      | end
  Constant : Constant  Value=0
  Demux : Demux
  Display1 : Display
  Display3 : Display
  Heading Indicator1 : Subsystem  DialogController=aeroblksHMICreateDDGDialog  IsWebBlock=on  mask(MWDashboardBlock){webBlockId=70cbff24-c9d3-49dd-a244-2b87c077a69d, webBlockType=headingindicator, ShowInLibBrowser=on, ShowInitialText=on, HMISrcModelName=main}
      mask prompts: webBlockId "WebBlock Id"; webBlockType "WebBlock Type"; HMISrcModelName "Source Model"
      mask help: aeroblksHMI:aeroblkhmi:HeadingIndicatorDialogDesc
      mask Help: eval('asbhmihelp(''headingindicator'')');
      mask Display:
      | if strcmp(get_param(bdroot(gcb),'BlockDiagramType'), 'library')
      |  image([(matlabroot) '/toolbox/aeroblks/aeroblks/hmi/icons/HeadingIndicatorIcon.svg'])
      | end
  If : If  IfExpression=u1 == 1  ShowElse=off
  If Action Subsystem : Subsystem  TreatAsAtomicUnit=on
  Manual Switch : ManualSwitch
  Remaining Capacity Indicator1 : Subsystem  DialogController=hmiCreateDDGDialog  IsWebBlock=on  mask(MWDashboardBlock){webBlockId=33a1d8b9-32a8-419a-82d6-4d8c644b0d93, webBlockType=semicirculargauge, ShowInLibBrowser=on, ShowInitialText=on, HMISrcModelName=main}
      mask prompts: webBlockId "WebBlock Id"; webBlockType "WebBlock Type"; HMISrcModelName "Source Model"
      mask help: SimulinkHMI:dialogs:SemicircularGaugeDialogDesc
      mask Help: helpview([docroot '/mapfiles/simulink.map'], 'hmi_half_gauge')
      mask Display:
      | if strcmp(get_param(bdroot(gcb),'BlockDiagramType'), 'library')
      |     image([(matlabroot) '/toolbox/simulink/hmi/icons/SemicircularGauge.png']);
      | end
  Selector : Selector  IndexOptions=Index vector (dialog)  Indices=[1 2 3 4]  OutputSizes=1
  Selector1 : Selector  IndexOptions=Index vector (dialog)  Indices=[1 2 3 4 5 6 7 8 9 10 11 12]  OutputSizes=1
  Signal Builder : Subsystem  Tag=STV Subsys  LoadFcn=sigbuilder_block('load');  StartFcn=sigbuilder_block('start');  StopFcn=sigbuilder_block('stop');  ClipboardFcn=sigbuilder_block('clipboard');  mask(Sigbuilder block){tuvar=[0:10]}
      mask help: Simulink:masks:SigbuilderBlock_MD
      mask init:
      | if ~strcmp(get_param(bdroot(gcbh),'SimulationStatus'),'stopped') tuvar = sigbuilder_block('maskInit'); end
      settings: CopyFcn=sigbuilder_block('copy');  DeleteFcn=sigbuilder_block('delete');  ModelCloseFcn=sigbuilder_block('modelClose');  PreSaveFcn=sigbuilder_block('preSave');  PauseFcn=sigbuilder_block('pause');  ContinueFcn=sigbuilder_block('continue');  NameChangeFcn=sigbuilder_block('namechange');  OpenFcn=sigbuilder_block('open',[474 99 960 647.25 ]);  CloseFcn=sigbuilder_block('close');
      mask Display: plot(0, 0, 100, 100,[2, 2, 32, 32, 2], [68, 8, 8, 68, 68],[32, 2], [38, 38], [32, 19, 2],[53, 60, 44], [32, 17, 17, 2],[16, 16, 31, 31]);txt = getActiveGroup(gcbh);text(2, 100, txt,'verticalAlignment', 'top');
  Switch : Switch  Criteria=u2 > Threshold
  Terminator : Terminator
  d : Constant  Value=80
  flightCondition : Constant  Value=0
  PilotCmd : Outport  OutDataTypeStr=Bus: CommandBus
  wires:
  Signal Builder/1(Roll) -> Bus Creator/1  "roll_cmd"
  Signal Builder/2(Pitch) -> Bus Creator/2  "pitch_cmd"
  Signal Builder/3(Yaw) -> Bus Creator/3  "yaw_cmd"
  Manual Switch/1 -> Bus Creator/4  "altitude_cmd"
  Signal Builder/5(Throttle1) -> Bus Creator1/5, Bus Creator/5  "Throttle1_cmd"
  Bus Creator/1 -> Switch/3
  Switch/1 -> PilotCmd/1
  flightCondition/1 -> Bus Creator1/6, Bus Creator/6  "flightCondition"
  0/1 -> Bus Creator/7, Bus Creator1/7  "Position_cmd"
  Bus Creator1/1 -> Switch/1
  If Action Subsystem/1(Axes) -> Selector/1  "axes"
  Demux/1 -> Bus Creator1/1  "roll_cmd"
  Demux/4 -> Bus Creator1/4  "altitude_cmd"
  Demux/2 -> Bus Creator1/2  "pitch_cmd"
  Demux/3 -> Bus Creator1/3  "yaw_cmd"
  If Action Subsystem/2(Buttons) -> Selector1/1  "buttons"
  Buttons to Switches/1(Switches) -> Display3/1
  Constant/1 -> [joystickEnable], Bus Creator/8, Bus Creator1/8, Switch/2  "joystickEnabled"
  Selector1/1 -> Display1/1, Buttons to Switches/1(Buttons)
  Selector/1 -> Demux/1
  Signal Builder/6(flightCondition) -> Terminator/1  "flightCondition"
  [joystickEnable] -> If/1
  If/1 -> If Action Subsystem/Action
  Signal Builder/4(Altitude) -> Manual Switch/2  "altitude_cmd"
  d/1 -> Manual Switch/1

== system main/Sensors ==
  note: 1) Add Subsystem or Model blocks as valid variant choices.
      | 2) You cannot connect blocks at this level. At simulation, connectivity is automatically
      | determined, based on the active variant and port name matching.
  Environment : Inport  OutDataTypeStr=Bus: envDataBus
  States : Inport  Port=2  OutDataTypeStr=Bus: plantDataBus
  Feedthrough Sensors : Subsystem  VariantControl=noisySensors~=1
  Noisy Sensors : Subsystem  VariantControl=noisySensors==1
  Sensors : Outport  OutDataTypeStr=Bus: SensorsBus

== system main/Visualization ==
  States : Inport  OutDataTypeStr=Bus: plantDataBus
  Commands : Inport  Port=2  OutDataTypeStr=Bus: CommandBus
  Airspeed Indicator : Subsystem  DialogController=aeroblksHMICreateDDGDialog  IsWebBlock=on  mask(MWDashboardBlock){webBlockId=1660c180-4922-4edc-b12a-b6c4fb3472e7, webBlockType=airspeedindicator, ShowInLibBrowser=on, ShowInitialText=on, HMISrcModelName=main}
      mask prompts: webBlockId "WebBlock Id"; webBlockType "WebBlock Type"; HMISrcModelName "Source Model"
      mask help: aeroblksHMI:aeroblkhmi:AirspeedIndicatorDialogDesc
      mask Help: eval('asbhmihelp(''airspeedindicator'')');
      mask Display:
      | if strcmp(get_param(bdroot(gcb),'BlockDiagramType'), 'library')
      |  image([(matlabroot) '/toolbox/aeroblks/aeroblks/hmi/icons/AirspeedIndicatorIcon.svg'])
      | end
  Alpha and beta visualization : Scope  NumInputPorts=2
  Altimeter : Subsystem  DialogController=aeroblksHMICreateDDGDialog  IsWebBlock=on  mask(MWDashboardBlock){webBlockId=dac4b64b-8b08-4b88-951c-85bcef5f9a8d, webBlockType=altimeter, ShowInLibBrowser=on, ShowInitialText=on, HMISrcModelName=main}
      mask prompts: webBlockId "WebBlock Id"; webBlockType "WebBlock Type"; HMISrcModelName "Source Model"
      mask help: aeroblksHMI:aeroblkhmi:AltimeterDialogDesc
      mask Help: eval('asbhmihelp(''altimeter'')');
      mask Display:
      | if strcmp(get_param(bdroot(gcb),'BlockDiagramType'), 'library')
      |  image([(matlabroot) '/toolbox/aeroblks/aeroblks/hmi/icons/AltimeterIcon.svg'])
      | end
  Altitude : Scope
  Artificial Horizon : Subsystem  DialogController=aeroblksHMICreateDDGDialog  IsWebBlock=on  mask(MWDashboardBlock){webBlockId=71b89583-386f-4e5a-a87e-fbc6faf0c9b0, webBlockType=artificialhorizon, ShowInLibBrowser=on, ShowInitialText=on, HMISrcModelName=main}
      mask prompts: webBlockId "WebBlock Id"; webBlockType "WebBlock Type"; HMISrcModelName "Source Model"
      mask help: aeroblksHMI:aeroblkhmi:ArtificialHorizonDialogDesc
      mask Help: eval('asbhmihelp(''artificialhorizon'')');
      mask Display:
      | if strcmp(get_param(bdroot(gcb),'BlockDiagramType'), 'library')
      |  image([(matlabroot) '/toolbox/aeroblks/aeroblks/hmi/icons/ArtificialHorizonIcon.svg'])
      | end
  Axes to VR Axes : Subsystem
  Bus Selector : BusSelector  OutputSignals=X_ned
  Bus Selector1 : BusSelector  OutputSignals=Euler.phi,Euler.theta,Euler.psi
  Bus Selector2 : BusSelector  OutputSignals=LLA.Altitude_m
  Bus Selector3 : BusSelector  OutputSignals=V_body,V_ned
  Bus Selector4 : BusSelector  OutputSignals=alpha,beta
  Bus Selector5 : BusSelector  OutputSignals=LLA.Latitude_deg,LLA.Longitude_deg
  Bus Selector6 : BusSelector  OutputSignals=remainingCapacity
  Climb Rate Indicator : Subsystem  DialogController=aeroblksHMICreateDDGDialog  IsWebBlock=on  mask(MWDashboardBlock){webBlockId=2290786a-142e-4cdc-9e89-cbe88d1b2ef4, webBlockType=climbindicator, ShowInLibBrowser=on, ShowInitialText=on, HMISrcModelName=main}
      mask prompts: webBlockId "WebBlock Id"; webBlockType "WebBlock Type"; HMISrcModelName "Source Model"
      mask help: aeroblksHMI:aeroblkhmi:ClimbIndicatorDialogDesc
      mask Help: eval('asbhmihelp(''climbindicator'')');
      mask Display:
      | if strcmp(get_param(bdroot(gcb),'BlockDiagramType'), 'library')
      |  image([(matlabroot) '/toolbox/aeroblks/aeroblks/hmi/icons/ClimbIndicatorIcon.svg'])
      | end
  Demux : Demux  Outputs=3
  Demux1 : Demux  Outputs=3
  Demux2 : Demux  Outputs=3
  Earth position : Scope  NumInputPorts=3
  Euler angles visualization : Scope  NumInputPorts=3
  Gain : Gain  Gain=-1
  Heading Indicator : Subsystem  DialogController=aeroblksHMICreateDDGDialog  IsWebBlock=on  mask(MWDashboardBlock){webBlockId=f0aafb45-9505-4aed-89ac-b6a93bae7c37, webBlockType=headingindicator, ShowInLibBrowser=on, ShowInitialText=on, HMISrcModelName=main}
      mask prompts: webBlockId "WebBlock Id"; webBlockType "WebBlock Type"; HMISrcModelName "Source Model"
      mask help: aeroblksHMI:aeroblkhmi:HeadingIndicatorDialogDesc
      mask Help: eval('asbhmihelp(''headingindicator'')');
      mask Display:
      | if strcmp(get_param(bdroot(gcb),'BlockDiagramType'), 'library')
      |  image([(matlabroot) '/toolbox/aeroblks/aeroblks/hmi/icons/HeadingIndicatorIcon.svg'])
      | end
  Mux : Mux  Inputs=3
  Mux3 : Mux  Inputs=3
  Rate Transition : RateTransition  Commented=through
  Rate Transition1 : RateTransition  Commented=through
  Remaining Capacity Indicator : Subsystem  DialogController=hmiCreateDDGDialog  IsWebBlock=on  mask(MWDashboardBlock){webBlockId=3cc98715-4e0e-4af5-a1de-baf30d0f48a0, webBlockType=semicirculargauge, ShowInLibBrowser=on, ShowInitialText=on, HMISrcModelName=main}
      mask prompts: webBlockId "WebBlock Id"; webBlockType "WebBlock Type"; HMISrcModelName "Source Model"
      mask help: SimulinkHMI:dialogs:SemicircularGaugeDialogDesc
      mask Help: helpview([docroot '/mapfiles/simulink.map'], 'hmi_half_gauge')
      mask Display:
      | if strcmp(get_param(bdroot(gcb),'BlockDiagramType'), 'library')
      |     image([(matlabroot) '/toolbox/simulink/hmi/icons/SemicircularGauge.png']);
      | end
  Rotation Angles to Direction Cosine Matrix : aerolibtransform2/Rotation Angles to Direction Cosine Matrix  rotationOrder=ZXY
  Rotation Matrix to VRML Rotation : vrlib/Utilities/Rotation Matrix to VRML Rotation  maxzero=1e-12
  Scope : Scope  NumInputPorts=2
  Subsystem : Subsystem
  Terminator{,1..6} (7 alike) : Terminator
  VR Sink : vrlib/VR Sink  InstantiateOnLoad=on  SampleTime=-1  ViewEnable=on  RemoteChange=off  RemoteView=off  FieldsWritten=Plane.rotation.4.1.1.double#Plane.translation.3.1.1.double  WorldFileName=\graphics\vr.wrl  WorldDescription=VR Plane Take-Off  AutoView=on  VideoDimensions=[]  AllowVariableSize=off  FigureProperties="{'Position', 'Name', 'Viewpoint', 'CameraBound', 'CameraDirection', 'CameraPosition', 'CameraUpVector', 'ZoomFactor', 'Antialiasing', 'Headlight', 'Lighting', 'NavPanel', 'Sound', 'StatusBar', 'Stereo3D', 'Stereo3DCameraOffset', 'Stereo3DHIT', 'ToolBar', 'Textures', 'Transparency', 'Triad', 'Wireframe', 'NavZones', 'NavMode', 'NavSpeed', 'CaptureFileFormat', 'CaptureFileName', 'Record2DCompressMethod', 'Record2DCompressQuality', 'Record2D', 'Record2DFileName', 'Record2DFPS'; [1.0520000000000000e+03   4.6000000000000000e+02   5.2600000000000000e+02   3.4100000000000000e+02], 'VR Plane Take-Off', 'See Whole Trajectory', 'on', [2.6780040025109136e-01  -2.2175423343042688e-01  -9.3760759680211447e-01], [3.5763663384731830e+00  -1.5808540570134588e+00  -1.6466435396223435e+01], [1.9863103344942779e-02   9.7421645617211750e-01  -2.2473930152277091e-01], [1.0000000000000000e+00], 'on', 'on', 'on', 'halfbar', 'on', 'on', 'off', [1.0000000149011612e-01], [0.0000000000000000e+00], 'on', 'on', 'on', 'none', 'off', 'off', 'fly', 'normal', 'tif', '%f_anim_%n.tif', 'auto', [7.5000000000000000e+01], 'off', '%f_anim_%n.avi', 'auto'}"  mask(Virtual Reality Sink){}
      mask Display:
      | % This is a new mask on top of the base mask.
      | % Use "View base mask" link below to see the base mask.
      | imageName='vr.wrl.thumbnail.png';
      | currentPath=get_param(bdroot, 'FileName');
      | positions=strfind(currentPath,'\');
      | imagePath=strcat(currentPath(1:positions(end-1)),'graphics\',imageName);
      | image(imagePath);
  V_body visualization : Scope  NumInputPorts=3
  V_ned visualization : Scope  NumInputPorts=3
  wires:
  Bus Selector1/1 -> Euler angles visualization/1, Mux/1, Gain/1  "<phi>"
  Bus Selector1/2 -> Mux/2, Mux3/2, Euler angles visualization/2  "<theta>"
  Bus Selector1/3 -> Mux/3, Mux3/3, Euler angles visualization/3  "<psi>"
  States/1 -> Bus Selector/1, Bus Selector1/1, Bus Selector5/1, Bus Selector6/1, Bus Selector4/1, Bus Selector3/1, Bus Selector2/1
  Bus Selector2/1 -> Altitude/1  "<Altitude_m>"
  Axes to VR Axes/1(Xe VR) -> Rate Transition1/1
  Bus Selector/1 -> Demux/1, Subsystem/1("X_ned "), Axes to VR Axes/1(Xe)  "<X_ned>"
  Mux/1 -> Subsystem/2(Euler_angles)  "Euler Angles"
  Bus Selector3/1 -> Subsystem/3(V_body), Demux2/1  "<V_body>"
  Bus Selector3/2 -> Subsystem/4(V_ned), Demux1/1  "<V_ned>"
  Subsystem/1(Airspeed (kts)) -> Terminator/1
  Subsystem/2(Height (ft)) -> Terminator1/1
  Subsystem/3(Roll Flightpath (deg)) -> Terminator2/1
  Subsystem/4(Climb Rate (ft/min)) -> Terminator3/1
  Subsystem/5(Heading (deg)) -> Terminator4/1
  Demux/2 -> Earth position/2
  Demux/1 -> Earth position/1
  Demux/3 -> Earth position/3
  Bus Selector4/1 -> Alpha and beta visualization/1  "<alpha>"
  Bus Selector4/2 -> Alpha and beta visualization/2  "<beta>"
  Demux1/1 -> V_ned visualization/1  "V_ned_x"
  Demux1/2 -> V_ned visualization/2  "V_ned_y"
  Demux1/3 -> V_ned visualization/3  "V_ned_z"
  Demux2/1 -> V_body visualization/1  "V_body_x"
  Demux2/2 -> V_body visualization/2  "V_body_y"
  Demux2/3 -> V_body visualization/3  "V_body_z"
  Commands/1 -> Terminator5/1
  Bus Selector5/1 -> Scope/1  "<Latitude_deg>"
  Bus Selector5/2 -> Scope/2  "<Longitude_deg>"
  Bus Selector6/1 -> Terminator6/1  "<remainingCapacity>"
  Rotation Matrix to VRML Rotation/1 -> Rate Transition/1
  Rotation Angles to Direction Cosine Matrix/1 -> Rotation Matrix to VRML Rotation/1
  Mux3/1 -> Rotation Angles to Direction Cosine Matrix/1
  Gain/1 -> Mux3/1
  Rate Transition/1 -> VR Sink/1  "rotation"
  Rate Transition1/1 -> VR Sink/2  "translation"

== system main/Actuators/Feedthrough ==
  ActuatorsCmd : Inport  OutDataTypeStr=Bus: ActuatorsBus
  Actuators : Outport  OutDataTypeStr=Bus: ActuatorsBus
  wires:
  ActuatorsCmd/1 -> Actuators/1

== system main/Actuators/Linear 1st Order ==
  ActuatorsCmd : Inport  OutDataTypeStr=Bus: ActuatorsBus
  Bus Creator : BusCreator  Inputs='deltae','deltar','deltafr','deltafl'  OutDataTypeStr=Bus: ActuatorsBus  NonVirtualBus=on
  Bus Selector : BusSelector  OutputSignals=deltae,deltar,deltafr,deltafl
  deltae : TransferFcn  Numerator=[a]  Denominator=[1 a]
  deltaefl : TransferFcn  Numerator=[a]  Denominator=[1 a]
  deltafr : TransferFcn  Numerator=[a]  Denominator=[1 a]
  deltar : TransferFcn  Numerator=[a]  Denominator=[1 a]
  Actuators : Outport  OutDataTypeStr=Bus: ActuatorsBus
  wires:
  Bus Creator/1 -> Actuators/1  "Actuators"
  deltafr/1 -> Bus Creator/3  "deltafr"
  Bus Selector/3 -> deltafr/1  "<deltafr>"
  Bus Selector/4 -> deltaefl/1  "<deltafl>"
  deltar/1 -> Bus Creator/2  "deltar"
  Bus Selector/2 -> deltar/1  "<deltar>"
  deltae/1 -> Bus Creator/1  "deltae"
  Bus Selector/1 -> deltae/1  "<deltae>"
  deltaefl/1 -> Bus Creator/4  "deltafl"
  ActuatorsCmd/1 -> Bus Selector/1

== system main/Actuators/Linear 2nd Order ==
  ActuatorsCmd : Inport  OutDataTypeStr=Bus: ActuatorsBus
  Linear Second-Order Actuator : aerolibactuator/Linear Second-Order Actuator  wn_fin=LD.Actuators.LSO.naturalFreq  z_fin=LD.Actuators.LSO.dampingRatio  fin_act_0=LD.Actuators.LSO.initialPosition  fin_act_vel=LD.Actuators.LSO.initialVelocity
  Actuators : Outport  OutDataTypeStr=Bus: ActuatorsBus
  wires:
  ActuatorsCmd/1 -> Linear Second-Order Actuator/1
  Linear Second-Order Actuator/1 -> Actuators/1

== system main/Actuators/Nonlinear 2nd Order ==
  ActuatorsCmd : Inport  OutDataTypeStr=Bus: ActuatorsBus
  Nonlinear Second-Order Actuator : aerolibactuator/Nonlinear Second-Order Actuator  wn_fin=LD.Actuators.NLSO.naturalFreq  z_fin=LD.Actuators.NLSO.dampingRatio  fin_max=LD.Actuators.NLSO.maxDeflection  fin_min=LD.Actuators.NLSO.minDeflection  fin_maxrate=LD.Actuators.NLSO.rateLimit  fin_act_0=LD.Actuators.NLSO.initialPosition  fin_act_vel=LD.Actuators.NLSO.initialVelocity
  Actuators : Outport  OutDataTypeStr=Bus: ActuatorsBus
  wires:
  Nonlinear Second-Order Actuator/1 -> Actuators/1
  ActuatorsCmd/1 -> Nonlinear Second-Order Actuator/1
